simulink model "test1"  (Simulink 9.3)
settings: Solver=VariableStepAuto  StartTime=0.0  StopTime=200  RelTol=1e-3  EnableMultiTasking=on
settings Model: Creator=HLQ  LastModifiedBy=Administrator
settings DataIOCC: LimitDataPoints=on  SignalLoggingSaveFormat=Dataset
settings DebuggingCC: UnderspecifiedInitializationDetection=Simplified  MergeDetectMultiDrivingBlocksExec=error  SolverPrmCheckMsg=warning  FcnCallInpInsideContextMsg=error
settings GRTTargetCC: GeneratePreprocessorConditionals=Disable all  CombineOutputUpdateFcns=on  GRTInterface=off
settings ConfigComp: CovSFcnEnable=off

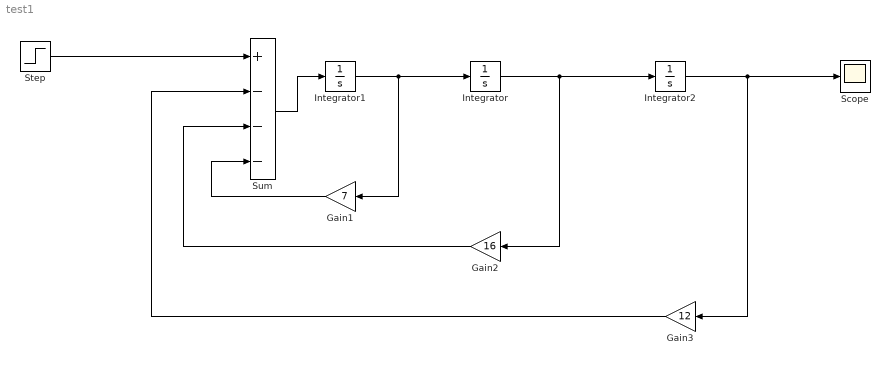
== system test1 ==
  Gain1 : Gain  Gain=7
  Gain2 : Gain  Gain=16
  Gain3 : Gain  Gain=12
  Integrator : Integrator
  Integrator1 : Integrator
  Integrator2 : Integrator
  Scope : Scope
  Step : Step  SampleTime=0
  Sum : Sum  Inputs=+---
  wires:
  Integrator1/1 -> Gain1/1, Integrator/1
  Integrator/1 -> Gain2/1, Integrator2/1
  Sum/1 -> Integrator1/1
  Step/1 -> Sum/1
  Gain1/1 -> Sum/4
  Gain2/1 -> Sum/3
  Integrator2/1 -> Gain3/1, Scope/1
  Gain3/1 -> Sum/2
